simulink model "LimitChecker"  (Simulink 6.6)
settings: Solver=FixedStepDiscrete  SolverMode=SingleTasking  StartTime=0.0  StopTime=50  FixedStep=sample  RelTol=1e-3
undefined symbols (not defined in the file or in its folder): sample
settings Model: Creator=Tommy  LastModifiedBy=Tommy

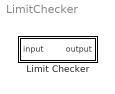
== system LimitChecker ==
  Limit Checker : Subsystem  mask{upperlimit=15, lowerlimit=-25}

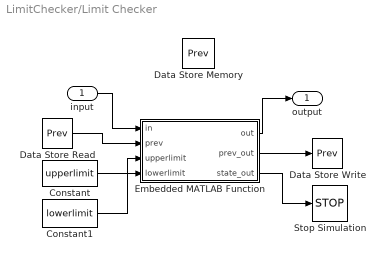
== system LimitChecker/Limit Checker ==
  input : Inport
  Constant : Constant  Value=upperlimit
  Constant1 : Constant  Value=lowerlimit
  Data Store Memory : DataStoreMemory  DataStoreName=Prev  InitialValue=0
  Data Store Read : DataStoreRead  DataStoreName=Prev  SampleTime=sample
  Data Store Write : DataStoreWrite  DataStoreName=Prev  SampleTime=-1
  Embedded MATLAB Function : Stateflow chart
  Stop Simulation : Stop
  output : Outport
  wires:
  Embedded MATLAB Function/3(state_out) -> Stop Simulation/1
  Embedded MATLAB Function/1(out) -> output/1
  input/1 -> Embedded MATLAB Function/1(in)
  Constant1/1 -> Embedded MATLAB Function/4(lowerlimit)
  Constant/1 -> Embedded MATLAB Function/3(upperlimit)
  Data Store Read/1 -> Embedded MATLAB Function/2(prev)
  Embedded MATLAB Function/2(prev_out) -> Data Store Write/1

== matlab function Limit Checker/Embedded MATLAB Function ==
  data: in input inherited; prev input inherited; out output inherited; prev_out output inherited; state_out output inherited; upperlimit input inherited; lowerlimit input inherited
function [out,prev_out,state_out] = fcn(in,prev,upperlimit,lowerlimit)

if ((in <= upperlimit) && (in >= lowerlimit))
    % ok
    out = in;
    prev_out = in;
    state_out = 0;
else
    % limit hit
    out = prev;
    prev_out = out;
    state_out = 1;
end
